simulink model "tmp_model_6"  (R2018b)
settings: Solver=ode15s  StartTime=0.0  StopTime=20  FixedStep=0.001  MaxStep=0.02  RelTol=1e-3
libraries: fl_lib x57, sdl_lib x18, powerlib_meascontrol x10, nesl_utility x9, simulink x2
(part 3 of 3)

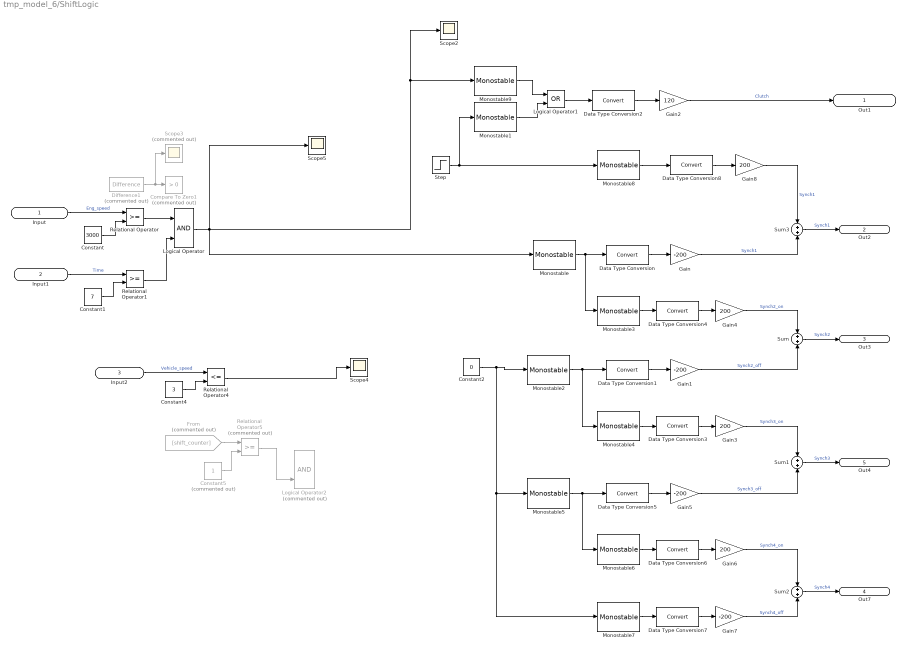
== system tmp_model_6/ShiftLogic ==
  Input : Inport
  Input1 : Inport  Port=2
  Input2 : Inport  Port=3
  Compare To Zero1 : simulink/Logic and Bit Operations/Compare To Zero  Commented=on  relop=>  OutDataTypeStr=boolean
  Constant : Constant  Value=3000
  Constant1 : Constant  Value=7
  Constant2 : Constant  Value=0
  Constant4 : Constant  Value=3
  Constant5 : Constant  Commented=on
  Data Type Conversion{,1..8} (9 alike) : DataTypeConversion
  Difference1 : simulink/Quick Insert/Discrete/Difference  Commented=on  ICPrevInput=0.0  OutMin=[]  OutMax=[]  OutDataType=fixdt(1, 16)  OutScaling=2^-10  DoSatur=off
      settings: SourceProductName=Simulink  SourceProductBaseCode=SL
  From : From  Commented=on  GotoTag=shift_counter
  Gain{,1,5,7} (4 alike) : Gain  Gain=-200
  Gain2 : Gain  Gain=120
  Gain{3..4,6,8} (4 alike) : Gain  Gain=200
  Logical Operator : Logic  AllPortsSameDT=off  OutDataTypeStr=boolean
  Logical Operator1 : Logic  Operator=OR  AllPortsSameDT=off  OutDataTypeStr=boolean
  Logical Operator2 : Logic  Commented=on  AllPortsSameDT=off  OutDataTypeStr=boolean
  Monostable{,2,5,7..8} (5 alike) : powerlib_meascontrol/Logic/Monostable  EdgeDetect=Rising  PulseDuration=1.5  ic=0  Ts=0
      settings: SourceProductName=Simscape Power Systems  SourceProductBaseCode=PS
  Monostable1 : powerlib_meascontrol/Logic/Monostable  EdgeDetect=Rising  PulseDuration=2  ic=0  Ts=0
      settings: SourceProductName=Simscape Power Systems  SourceProductBaseCode=PS
  Monostable3 : powerlib_meascontrol/Logic/Monostable  EdgeDetect=Falling  PulseDuration=1.5  ic=0  Ts=0
      settings: SourceProductName=Simscape Power Systems  SourceProductBaseCode=PS
  Monostable4 : powerlib_meascontrol/Logic/Monostable  EdgeDetect=Falling  PulseDuration=1.5  ic=0  Ts=0
      settings: SourceProductName=Simscape Power Systems  SourceProductBaseCode=PS
  Monostable6 : powerlib_meascontrol/Logic/Monostable  EdgeDetect=Falling  PulseDuration=1.5  ic=0  Ts=0
      settings: SourceProductName=Simscape Power Systems  SourceProductBaseCode=PS
  Monostable9 : powerlib_meascontrol/Logic/Monostable  EdgeDetect=Rising  PulseDuration=2  ic=0  Ts=0
      settings: SourceProductName=Simscape Power Systems  SourceProductBaseCode=PS
  Relational Operator : RelationalOperator  OutDataTypeStr=boolean  RndMeth=Simplest
  Relational Operator1 : RelationalOperator  OutDataTypeStr=boolean  RndMeth=Simplest
  Relational Operator4 : RelationalOperator  Operator=<=  OutDataTypeStr=boolean  RndMeth=Simplest
  Relational Operator5 : RelationalOperator  Commented=on  OutDataTypeStr=boolean  RndMeth=Simplest
  Scope2 : Scope
  Scope3 : Scope  Commented=on
  Scope4 : Scope
  Scope5 : Scope
  Step : Step  Time=0.5  SampleTime=0
  Sum{,1..3} (4 alike) : Sum  Inputs=+|+
  Out1 : Outport
  Out2 : Outport  Port=2
  Out3 : Outport  Port=3
  Out7 : Outport  Port=4
  Out4 : Outport  Port=5
  wires:
  Input/1 -> Relational Operator/1  "Eng_speed"
  Monostable/1 -> Data Type Conversion/1, Monostable3/1
  Monostable1/1 -> Logical Operator1/2
  Monostable3/1 -> Data Type Conversion4/1
  Data Type Conversion4/1 -> Gain4/1
  Constant/1 -> Relational Operator/2
  Constant1/1 -> Relational Operator1/2
  Data Type Conversion/1 -> Gain/1
  Input1/1 -> Relational Operator1/1  "Time"
  Difference1/1 -> Scope3/1, Compare To Zero1/1
  Data Type Conversion2/1 -> Gain2/1
  Gain2/1 -> Out1/1  "Clutch"
  Gain/1 -> Sum3/2  "Synch1"
  Gain4/1 -> Sum/1  "Synch2_on"
  Gain3/1 -> Sum1/1  "Synch3_on"
  Gain1/1 -> Sum/2  "Synch2_off"
  Data Type Conversion1/1 -> Gain1/1
  Data Type Conversion3/1 -> Gain3/1
  Monostable4/1 -> Data Type Conversion3/1
  Monostable2/1 -> Monostable4/1, Data Type Conversion1/1
  Monostable5/1 -> Data Type Conversion5/1, Monostable6/1
  Monostable6/1 -> Data Type Conversion6/1
  Data Type Conversion6/1 -> Gain6/1
  Data Type Conversion5/1 -> Gain5/1
  Gain5/1 -> Sum1/2  "Synch3_off"
  Gain6/1 -> Sum2/1  "Synch4_on"
  Input2/1 -> Relational Operator4/1  "Vehicle_speed"
  Constant4/1 -> Relational Operator4/2
  Sum/1 -> Out3/1  "Synch2"
  Sum1/1 -> Out4/1  "Synch3"
  Data Type Conversion7/1 -> Gain7/1
  Monostable7/1 -> Data Type Conversion7/1
  Gain7/1 -> Sum2/2  "Synch4_off"
  Sum2/1 -> Out7/1  "Synch4"
  Relational Operator/1 -> Logical Operator/1
  Relational Operator1/1 -> Logical Operator/2
  From/1 -> Relational Operator5/1
  Constant5/1 -> Relational Operator5/2
  Relational Operator5/1 -> Logical Operator2/2
  Relational Operator4/1 -> Scope4/1
  Constant2/1 -> Monostable7/1, Monostable5/1, Monostable2/1
  Data Type Conversion8/1 -> Gain8/1
  Monostable8/1 -> Data Type Conversion8/1
  Gain8/1 -> Sum3/1  "Synch1"
  Sum3/1 -> Out2/1  "Synch1"
  Logical Operator/1 -> Scope2/1, Monostable9/1, Monostable/1, Scope5/1
  Step/1 -> Monostable1/1, Monostable8/1
  Monostable9/1 -> Logical Operator1/1
  Logical Operator1/1 -> Data Type Conversion2/1

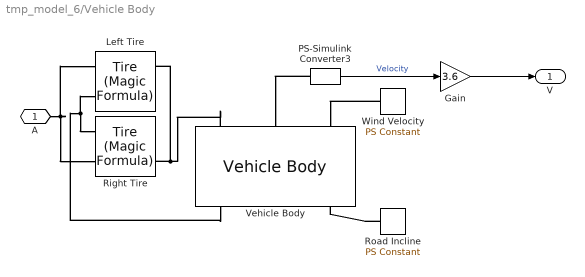
== system tmp_model_6/Vehicle Body ==
  Gain : Gain  Gain=3.6
  Left Tire : sdl_lib/Tires & Vehicles/Tire (Magic Formula)  parameterization=3  F_z1=3000 N  F_x1=3500 N  kappa1=10  B_m=10  C_m=1.9  D_m=1  E_m=0.97  fz0=4e+3 N  p_Cx=1.685  p_Dx=[ 1.21 -0.037 ]  p_Ex=[ 0.344 0.095 -0.02 0 ]  p_Kx=[ 21.51 -0.163 0.245 ]  p_Hx=[ -0.002 0.002 ]  p_Vx=[ 0 0 ]  v_tr_thr=0.1 m/s  r_e=0.685 m  model_compliance=0  stiffness=1e+6 N/m  damping=1000 N/(m/s)  model_inertia=1  inertia=0.8 kg*m^2  initial_velocity=0 rpm  model_resistance=0  resistance_model=1  coeff=0.015  p_tire=250e3 Pa  alpha=-0.003  beta=0.97  coeff_a=84e-4  coeff_b=6.2e-4 s/m  coeff_c=1.6e-4 s^2/m^2  v_thr=1e-3 m/s
      settings: SourceProductName=Simscape Driveline
  PS-Simulink Converter3 : nesl_utility/PS-Simulink Converter  PhysicalDomain=network_engine_domain  SubClassName=ps_output  LeftPortType=input  RightPortType=output  PseudoPeriodic=off  Frequencies=[]  Unit=m/s  AffineConversion=off
  Right Tire : sdl_lib/Tires & Vehicles/Tire (Magic Formula)  parameterization=3  F_z1=3000 N  F_x1=3500 N  kappa1=10  B_m=10  C_m=1.9  D_m=1  E_m=0.97  fz0=4e+3 N  p_Cx=1.685  p_Dx=[ 1.21 -0.037 ]  p_Ex=[ 0.344 0.095 -0.02 0 ]  p_Kx=[ 21.51 -0.163 0.245 ]  p_Hx=[ -0.002 0.002 ]  p_Vx=[ 0 0 ]  v_tr_thr=0.1 m/s  r_e=0.685 m  model_compliance=0  stiffness=1e+6 N/m  damping=1000 N/(m/s)  model_inertia=1  inertia=0.8 kg*m^2  initial_velocity=0 rpm  model_resistance=0  resistance_model=1  coeff=0.015  p_tire=250e3 Pa  alpha=-0.003  beta=0.97  coeff_a=84e-4  coeff_b=6.2e-4 s/m  coeff_c=1.6e-4 s^2/m^2  v_thr=1e-3 m/s
      settings: SourceProductName=Simscape Driveline
  Road Incline : fl_lib/Physical Signals/Sources/PS Constant  constant=0
  Vehicle Body : sdl_lib/Tires & Vehicles/Vehicle Body  mass=1200 kg  n_w=2  x_f=1.4 m  x_r=1.6 m  y_c=0.5 m  model_pitch=1  inertia=4000 kg*m^2  suspension_model=1  k_f=1e4 N/m  b_f=1e4 N/(m/s)  k_r=1e4 N/m  b_r=1e4 N/(m/s)  k_f_TLU=[-2000, -1000, 0, 1000, 2000] N  x_f_TLU=[-.4, -.2, 0, .2, .4] m  b_f_TLU=[-200, -100, 0, 100, 200] N  v_f_TLU=[-4, -2, 0, 2, 4] m/s  k_r_TLU=[-2000, -1000, 0, 1000, 2000] N  x_r_TLU=[-.4, -.2, 0, .2, .4] m  b_r_TLU=[-200, -100, 0, 100, 200] N  v_r_TLU=[-4, -2, 0, 2, 4] m/s  interp_method=simscape.enum.interpolation.linear  extrap_method=simscape.enum.extrapolation.linear  model_hardstop=0  upper_bound_f=.25 m  lower_bound_f=-.25 m  stop_k_f=1e6 N/m  stop_b_f=150 N/(m/s)  upper_bound_r=.25 m  lower_bound_r=-.25 m  stop_k_r=1e6 N/m  stop_b_r=150 N/(m/s)  initial_pitch=0 rad  initial_pitch_rate=0 rad/s  g=9.81 m/s^2  liftoff_warning=0  area=3 m^2  Cd=0.4  rho=1.18 kg/m^3  v_specify=on  v_priority=High  v=0 m/s  v_nominal_specify=off  v_nominal_unit=m/s  v_nominal_value=1
      settings: SourceProductName=Simscape Driveline
  Wind Velocity : fl_lib/Physical Signals/Sources/PS Constant  constant=0
  A : PMIOPort  Side=Left
  V : Outport
  wires:
  PS-Simulink Converter3/1 -> Gain/1  "Velocity"
  Gain/1 -> V/1
  connections:
  Right Tire/RConn2 -- Left Tire/RConn2 -- Vehicle Body/LConn1
  Vehicle Body/RConn1 -- Right Tire/LConn1 -- Left Tire/LConn1
  A/RConn1 -- Right Tire/LConn2 -- Left Tire/LConn2
  PS-Simulink Converter3/LConn1 -- Vehicle Body/LConn2
  Wind Velocity/RConn1 -- Vehicle Body/LConn3
  Road Incline/RConn1 -- Vehicle Body/RConn3

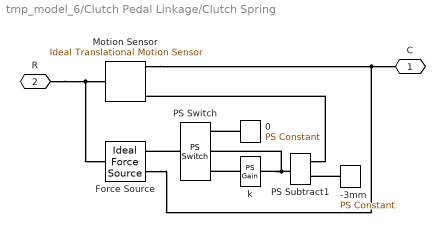
== system tmp_model_6/Clutch Pedal Linkage/Clutch Spring ==
  -3mm : fl_lib/Physical Signals/Sources/PS Constant  constant=-3e-3
  0 : fl_lib/Physical Signals/Sources/PS Constant  constant=0
  Force Source : fl_lib/Mechanical/Mechanical Sources/Ideal Force Source
  Motion Sensor : fl_lib/Mechanical/Mechanical Sensors/Ideal Translational Motion Sensor  offset=0 m
  PS Subtract1 : fl_lib/Physical Signals/Functions/PS Subtract
      settings: SourceProductName=Simscape
  PS Switch : fl_lib/Physical Signals/Nonlinear Operators/PS Switch  Threshold=0
      settings: SourceProductName=Simscape  SourceProductBaseCode=SS
  k : fl_lib/Physical Signals/Functions/PS Gain  gain=2000/3e-3
  C : PMIOPort  Side=Right
  R : PMIOPort  Port=2  Side=Left
  connections:
  -3mm/RConn1 -- PS Subtract1/LConn2
  Motion Sensor/RConn1 -- Force Source/RConn2 -- C/RConn1
  k/RConn1 -- PS Switch/LConn1
  PS Subtract1/LConn1 -- Motion Sensor/RConn3
  0/RConn1 -- PS Switch/LConn3
  R/RConn1 -- Motion Sensor/LConn1 -- Force Source/LConn1
  PS Subtract1/RConn1 -- PS Switch/LConn2 -- k/LConn1
  PS Switch/RConn1 -- Force Source/RConn1

== system tmp_model_6/GearBox/Gearbox Schematic ==

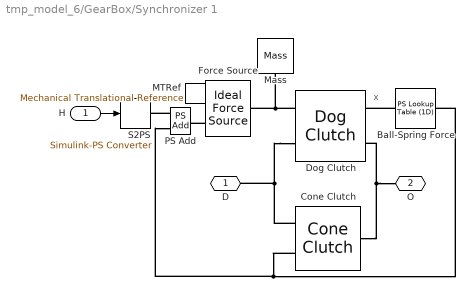
== system tmp_model_6/GearBox/Synchronizer 1 ==
  note: x
  H : Inport
  Ball-Spring Force : fl_lib/Physical Signals/Lookup Tables/PS Lookup Table (1D)  x=[ -2 -0.1 0 0.1 2 ]*1e-3+3.2e-3  f=[ 0 100 0 -100 0 ]  interp_method=1  extrap_method=2
      settings: SourceProductName=Simscape  SourceProductBaseCode=SS
  Cone Clutch : sdl_lib/Clutches/Cone Clutch  d_o=60 mm  d_i=50 mm  theta=15 deg  friction_model=1  mu_coulomb=0.5  mu_w_vector=[ 0 0.1 0.2 0.3 0.4 0.5 1 2 5 10 100 1000 ] rad/s  mu_coulomb_vector=[ 0.29 0.28 0.26 0.22 0.21 0.2 0.2 0.19 0.19 0.19 0.19 0.19 ]  mu_interp_method=1  mu_extrap_method=1  mu_static=0.52  w_tol=0.01 rad/s  force_min=1 N  initial_state_locked=0  temperature_TLU=[280.0, 300.0, 320.0] K  mu_coulomb_temp_vector=[0.3, 0.28, 0.25]  mu_coulomb_matrix=[0.34, 0.32, 0.3; 0.3, 0.28, 0.25; 0.25, 0.2, 0.15]  mu_static_vector=[0.4, 0.38, 0.36]  thermal_mass=25 kJ/K  T_init=300 K
      settings: SourceProductName=Simscape Driveline  SourceProductBaseCode=LD
  Dog Clutch : sdl_lib/Clutches/Dog Clutch  model=2  max_torque=1000 N*m  n_teeth=6  clutch_backlash=20 deg  tooth_height=10 mm  radius=50 mm  back_stop=1  ring_hub_gap=3 mm  clutch_stiffness=1e5 N*m/rad  clutch_damping=2000 N*m/(rad/s)  transl_stiffness=1e+7 N/m  transl_damping=1000 N/(m/s)  visc_fric_transl=10 N/(m/s)  fric_coeff=1e-7  direction=1  engagement_velocity=200 rpm  engagement_overlap=1 mm  initial_state_engaged=0  init_pos=0 mm  init_rel_angle=0 deg  temperature_TLU=[280.0, 300.0, 320.0] K  max_torque_vector=[1000.0, 1050.0, 1000.0] N*m  interp_method=1  extrap_method=1  thermal_mass=25 kJ/K  T_init=300 K
      settings: SourceProductName=Simscape Driveline  SourceProductBaseCode=LD
  Force Source : fl_lib/Mechanical/Mechanical Sources/Ideal Force Source
  MTRef : fl_lib/Mechanical/Translational Elements/Mechanical Translational Reference
  Mass : fl_lib/Mechanical/Translational Elements/Mass  mass=0.1 kg  v_specify=off  v_priority=High  v=0 m/s  v_nominal_specify=off  v_nominal_unit=m/s  v_nominal_value=1  f_specify=off  f_priority=High  f=0 N  f_nominal_specify=off  f_nominal_unit=N  f_nominal_value=1
  PS Add : fl_lib/Physical Signals/Functions/PS Add
  S2PS : nesl_utility/Simulink-PS Converter  PhysicalDomain=network_engine_domain  SubClassName=ps_input  LeftPortType=input  RightPortType=output  PseudoPeriodic=off  Frequencies=[]  NoiseDistribution=none  NoiseParameters=[]  Unit=1  AffineConversion=off  FilteringAndDerivatives=zero  SimscapeFilterOrder=1  InputFilterTimeConstant=.001  UdotUserProvided=1
  D : PMIOPort  Side=Left
  O : PMIOPort  Port=2  Side=Right
  wires:
  H/1 -> S2PS/1
  connections:
  Force Source/RConn1 -- PS Add/RConn1
  MTRef/LConn1 -- Force Source/RConn2
  Ball-Spring Force/LConn1 -- Dog Clutch/RConn1
  PS Add/LConn2 -- Ball-Spring Force/RConn1 -- Cone Clutch/LConn1
  O/RConn1 -- Dog Clutch/RConn2 -- Cone Clutch/RConn1
  Dog Clutch/LConn2 -- Cone Clutch/LConn2 -- D/RConn1
  Mass/LConn1 -- Force Source/LConn1 -- Dog Clutch/LConn1
  PS Add/LConn1 -- S2PS/RConn1

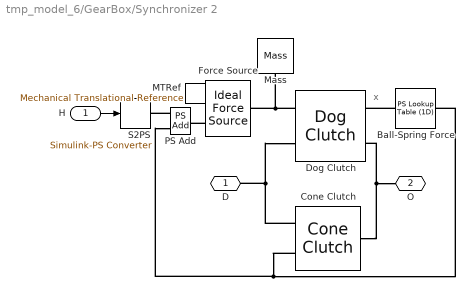
== system tmp_model_6/GearBox/Synchronizer 2 ==
  note: x
  H : Inport
  Ball-Spring Force : fl_lib/Physical Signals/Lookup Tables/PS Lookup Table (1D)  x=[ -2 -0.1 0 0.1 2 ]*1e-3+3.2e-3  f=[ 0 100 0 -100 0 ]  interp_method=1  extrap_method=2
      settings: SourceProductName=Simscape  SourceProductBaseCode=SS
  Cone Clutch : sdl_lib/Clutches/Cone Clutch  d_o=60 mm  d_i=50 mm  theta=15 deg  friction_model=1  mu_coulomb=0.5  mu_w_vector=[ 0 0.1 0.2 0.3 0.4 0.5 1 2 5 10 100 1000 ] rad/s  mu_coulomb_vector=[ 0.29 0.28 0.26 0.22 0.21 0.2 0.2 0.19 0.19 0.19 0.19 0.19 ]  mu_interp_method=1  mu_extrap_method=1  mu_static=0.52  w_tol=0.01 rad/s  force_min=1 N  initial_state_locked=0  temperature_TLU=[280.0, 300.0, 320.0] K  mu_coulomb_temp_vector=[0.3, 0.28, 0.25]  mu_coulomb_matrix=[0.34, 0.32, 0.3; 0.3, 0.28, 0.25; 0.25, 0.2, 0.15]  mu_static_vector=[0.4, 0.38, 0.36]  thermal_mass=25 kJ/K  T_init=300 K
      settings: SourceProductName=Simscape Driveline  SourceProductBaseCode=LD
  Dog Clutch : sdl_lib/Clutches/Dog Clutch  model=2  max_torque=1000 N*m  n_teeth=6  clutch_backlash=20 deg  tooth_height=10 mm  radius=50 mm  back_stop=1  ring_hub_gap=3 mm  clutch_stiffness=1e5 N*m/rad  clutch_damping=2000 N*m/(rad/s)  transl_stiffness=1e+7 N/m  transl_damping=1000 N/(m/s)  visc_fric_transl=10 N/(m/s)  fric_coeff=1e-7  direction=1  engagement_velocity=200 rpm  engagement_overlap=1 mm  initial_state_engaged=0  init_pos=0 mm  init_rel_angle=0 deg  temperature_TLU=[280.0, 300.0, 320.0] K  max_torque_vector=[1000.0, 1050.0, 1000.0] N*m  interp_method=1  extrap_method=1  thermal_mass=25 kJ/K  T_init=300 K
      settings: SourceProductName=Simscape Driveline  SourceProductBaseCode=LD
  Force Source : fl_lib/Mechanical/Mechanical Sources/Ideal Force Source
  MTRef : fl_lib/Mechanical/Translational Elements/Mechanical Translational Reference
  Mass : fl_lib/Mechanical/Translational Elements/Mass  mass=0.1 kg  v_specify=off  v_priority=High  v=0 m/s  v_nominal_specify=off  v_nominal_unit=m/s  v_nominal_value=1  f_specify=off  f_priority=High  f=0 N  f_nominal_specify=off  f_nominal_unit=N  f_nominal_value=1
  PS Add : fl_lib/Physical Signals/Functions/PS Add
  S2PS : nesl_utility/Simulink-PS Converter  PhysicalDomain=network_engine_domain  SubClassName=ps_input  LeftPortType=input  RightPortType=output  PseudoPeriodic=off  Frequencies=[]  NoiseDistribution=none  NoiseParameters=[]  Unit=1  AffineConversion=off  FilteringAndDerivatives=zero  SimscapeFilterOrder=1  InputFilterTimeConstant=.001  UdotUserProvided=1
  D : PMIOPort  Side=Left
  O : PMIOPort  Port=2  Side=Right
  wires:
  H/1 -> S2PS/1
  connections:
  PS Add/LConn1 -- S2PS/RConn1
  Dog Clutch/LConn1 -- Mass/LConn1 -- Force Source/LConn1
  Cone Clutch/LConn2 -- D/RConn1 -- Dog Clutch/LConn2
  Cone Clutch/RConn1 -- Dog Clutch/RConn2 -- O/RConn1
  Cone Clutch/LConn1 -- PS Add/LConn2 -- Ball-Spring Force/RConn1
  Ball-Spring Force/LConn1 -- Dog Clutch/RConn1
  MTRef/LConn1 -- Force Source/RConn2
  Force Source/RConn1 -- PS Add/RConn1

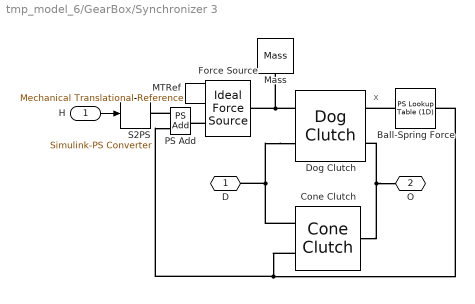
== system tmp_model_6/GearBox/Synchronizer 3 ==
  note: x
  H : Inport
  Ball-Spring Force : fl_lib/Physical Signals/Lookup Tables/PS Lookup Table (1D)  x=[ -2 -0.1 0 0.1 2 ]*1e-3+3.2e-3  f=[ 0 100 0 -100 0 ]  interp_method=1  extrap_method=2
      settings: SourceProductName=Simscape  SourceProductBaseCode=SS
  Cone Clutch : sdl_lib/Clutches/Cone Clutch  d_o=60 mm  d_i=50 mm  theta=15 deg  friction_model=1  mu_coulomb=0.5  mu_w_vector=[ 0 0.1 0.2 0.3 0.4 0.5 1 2 5 10 100 1000 ] rad/s  mu_coulomb_vector=[ 0.29 0.28 0.26 0.22 0.21 0.2 0.2 0.19 0.19 0.19 0.19 0.19 ]  mu_interp_method=1  mu_extrap_method=1  mu_static=0.52  w_tol=0.01 rad/s  force_min=1 N  initial_state_locked=0  temperature_TLU=[280.0, 300.0, 320.0] K  mu_coulomb_temp_vector=[0.3, 0.28, 0.25]  mu_coulomb_matrix=[0.34, 0.32, 0.3; 0.3, 0.28, 0.25; 0.25, 0.2, 0.15]  mu_static_vector=[0.4, 0.38, 0.36]  thermal_mass=25 kJ/K  T_init=300 K
      settings: SourceProductName=Simscape Driveline  SourceProductBaseCode=LD
  Dog Clutch : sdl_lib/Clutches/Dog Clutch  model=2  max_torque=1000 N*m  n_teeth=6  clutch_backlash=20 deg  tooth_height=10 mm  radius=50 mm  back_stop=1  ring_hub_gap=3 mm  clutch_stiffness=1e5 N*m/rad  clutch_damping=2000 N*m/(rad/s)  transl_stiffness=1e+7 N/m  transl_damping=1000 N/(m/s)  visc_fric_transl=10 N/(m/s)  fric_coeff=1e-7  direction=1  engagement_velocity=200 rpm  engagement_overlap=1 mm  initial_state_engaged=0  init_pos=0 mm  init_rel_angle=0 deg  temperature_TLU=[280.0, 300.0, 320.0] K  max_torque_vector=[1000.0, 1050.0, 1000.0] N*m  interp_method=1  extrap_method=1  thermal_mass=25 kJ/K  T_init=300 K
      settings: SourceProductName=Simscape Driveline  SourceProductBaseCode=LD
  Force Source : fl_lib/Mechanical/Mechanical Sources/Ideal Force Source
  MTRef : fl_lib/Mechanical/Translational Elements/Mechanical Translational Reference
  Mass : fl_lib/Mechanical/Translational Elements/Mass  mass=0.1 kg  v_specify=off  v_priority=High  v=0 m/s  v_nominal_specify=off  v_nominal_unit=m/s  v_nominal_value=1  f_specify=off  f_priority=High  f=0 N  f_nominal_specify=off  f_nominal_unit=N  f_nominal_value=1
  PS Add : fl_lib/Physical Signals/Functions/PS Add
  S2PS : nesl_utility/Simulink-PS Converter  PhysicalDomain=network_engine_domain  SubClassName=ps_input  LeftPortType=input  RightPortType=output  PseudoPeriodic=off  Frequencies=[]  NoiseDistribution=none  NoiseParameters=[]  Unit=1  AffineConversion=off  FilteringAndDerivatives=zero  SimscapeFilterOrder=1  InputFilterTimeConstant=.001  UdotUserProvided=1
  D : PMIOPort  Side=Left
  O : PMIOPort  Port=2  Side=Right
  wires:
  H/1 -> S2PS/1
  connections:
  Force Source/RConn1 -- PS Add/RConn1
  MTRef/LConn1 -- Force Source/RConn2
  Ball-Spring Force/LConn1 -- Dog Clutch/RConn1
  Ball-Spring Force/RConn1 -- PS Add/LConn2 -- Cone Clutch/LConn1
  O/RConn1 -- Dog Clutch/RConn2 -- Cone Clutch/RConn1
  Dog Clutch/LConn2 -- D/RConn1 -- Cone Clutch/LConn2
  Force Source/LConn1 -- Mass/LConn1 -- Dog Clutch/LConn1
  PS Add/LConn1 -- S2PS/RConn1

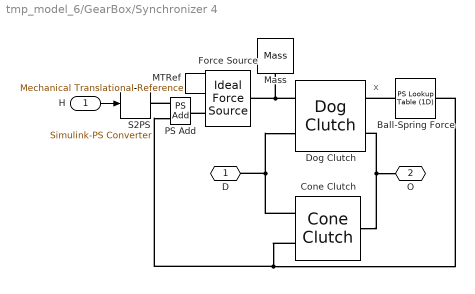
== system tmp_model_6/GearBox/Synchronizer 4 ==
  note: x
  H : Inport
  Ball-Spring Force : fl_lib/Physical Signals/Lookup Tables/PS Lookup Table (1D)  x=[ -2 -0.1 0 0.1 2 ]*1e-3+3.2e-3  f=[ 0 100 0 -100 0 ]  interp_method=1  extrap_method=2
      settings: SourceProductName=Simscape  SourceProductBaseCode=SS
  Cone Clutch : sdl_lib/Clutches/Cone Clutch  d_o=60 mm  d_i=50 mm  theta=15 deg  friction_model=1  mu_coulomb=0.5  mu_w_vector=[ 0 0.1 0.2 0.3 0.4 0.5 1 2 5 10 100 1000 ] rad/s  mu_coulomb_vector=[ 0.29 0.28 0.26 0.22 0.21 0.2 0.2 0.19 0.19 0.19 0.19 0.19 ]  mu_interp_method=1  mu_extrap_method=1  mu_static=0.52  w_tol=0.01 rad/s  force_min=1 N  initial_state_locked=0  temperature_TLU=[280.0, 300.0, 320.0] K  mu_coulomb_temp_vector=[0.3, 0.28, 0.25]  mu_coulomb_matrix=[0.34, 0.32, 0.3; 0.3, 0.28, 0.25; 0.25, 0.2, 0.15]  mu_static_vector=[0.4, 0.38, 0.36]  thermal_mass=25 kJ/K  T_init=300 K
      settings: SourceProductName=Simscape Driveline  SourceProductBaseCode=LD
  Dog Clutch : sdl_lib/Clutches/Dog Clutch  model=2  max_torque=1000 N*m  n_teeth=6  clutch_backlash=20 deg  tooth_height=10 mm  radius=50 mm  back_stop=1  ring_hub_gap=3 mm  clutch_stiffness=1e5 N*m/rad  clutch_damping=2000 N*m/(rad/s)  transl_stiffness=1e+7 N/m  transl_damping=1000 N/(m/s)  visc_fric_transl=10 N/(m/s)  fric_coeff=1e-7  direction=1  engagement_velocity=200 rpm  engagement_overlap=1 mm  initial_state_engaged=0  init_pos=0 mm  init_rel_angle=0 deg  temperature_TLU=[280.0, 300.0, 320.0] K  max_torque_vector=[1000.0, 1050.0, 1000.0] N*m  interp_method=1  extrap_method=1  thermal_mass=25 kJ/K  T_init=300 K
      settings: SourceProductName=Simscape Driveline  SourceProductBaseCode=LD
  Force Source : fl_lib/Mechanical/Mechanical Sources/Ideal Force Source
  MTRef : fl_lib/Mechanical/Translational Elements/Mechanical Translational Reference
  Mass : fl_lib/Mechanical/Translational Elements/Mass  mass=0.1 kg  v_specify=off  v_priority=High  v=0 m/s  v_nominal_specify=off  v_nominal_unit=m/s  v_nominal_value=1  f_specify=off  f_priority=High  f=0 N  f_nominal_specify=off  f_nominal_unit=N  f_nominal_value=1
  PS Add : fl_lib/Physical Signals/Functions/PS Add
  S2PS : nesl_utility/Simulink-PS Converter  PhysicalDomain=network_engine_domain  SubClassName=ps_input  LeftPortType=input  RightPortType=output  PseudoPeriodic=off  Frequencies=[]  NoiseDistribution=none  NoiseParameters=[]  Unit=1  AffineConversion=off  FilteringAndDerivatives=zero  SimscapeFilterOrder=1  InputFilterTimeConstant=.001  UdotUserProvided=1
  D : PMIOPort  Side=Left
  O : PMIOPort  Port=2  Side=Right
  wires:
  H/1 -> S2PS/1
  connections:
  PS Add/LConn1 -- S2PS/RConn1
  Dog Clutch/LConn1 -- Mass/LConn1 -- Force Source/LConn1
  Cone Clutch/LConn2 -- D/RConn1 -- Dog Clutch/LConn2
  Cone Clutch/RConn1 -- Dog Clutch/RConn2 -- O/RConn1
  Cone Clutch/LConn1 -- PS Add/LConn2 -- Ball-Spring Force/RConn1
  Ball-Spring Force/LConn1 -- Dog Clutch/RConn1
  MTRef/LConn1 -- Force Source/RConn2
  Force Source/RConn1 -- PS Add/RConn1
